simulink subsystem "tireTemp"  (R2022b)
settings: Solver=VariableStepAuto  StartTime=0.0  StopTime=10.0  RelTol=1e-3
libraries: tires x12
settings Model: Creator=serga  LastModifiedBy=serga

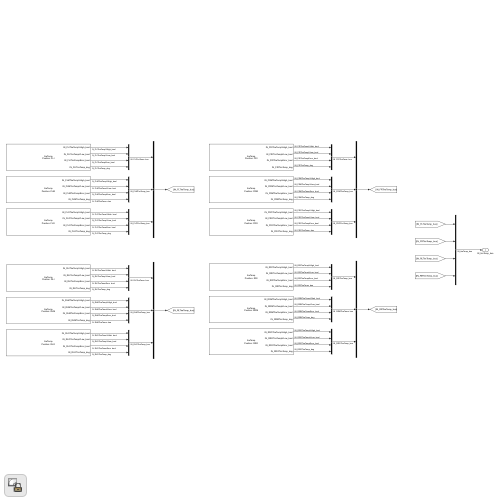
[thumbnail: Simulink's stored preview of the top-level diagram]
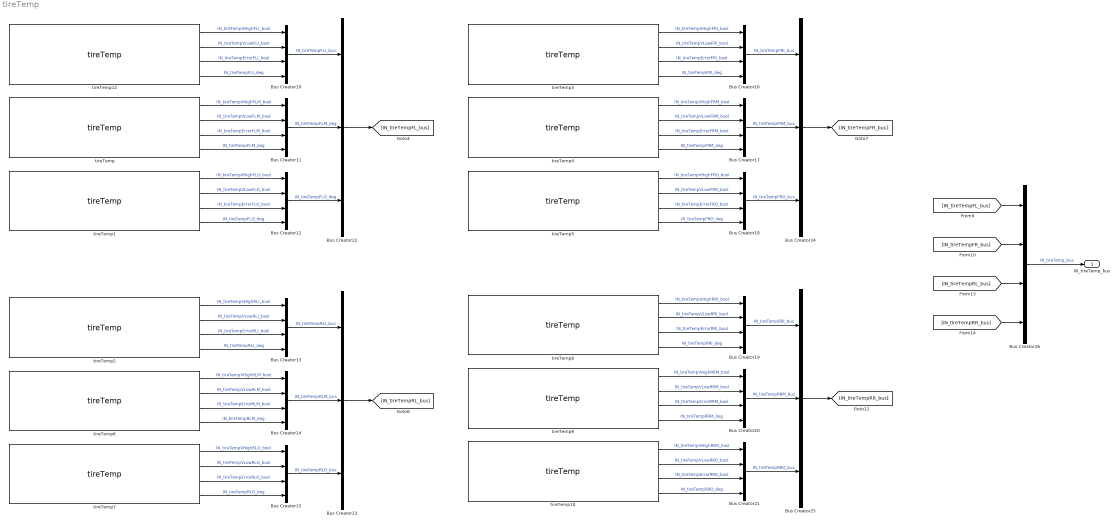
== system tireTemp ==
  Bus Creator{10..21,26} (13 alike) : BusCreator  Inputs=4
  Bus Creator{22..25} (4 alike) : BusCreator  Inputs=3
  tireTemp : tires/tireTemp  pos='FLM'
  tireTemp1 : tires/tireTemp  pos='FLO'
  tireTemp10 : tires/tireTemp  pos='RRO'
  tireTemp12 : tires/tireTemp  pos='FLI'
  tireTemp2 : tires/tireTemp  pos='RLI'
  tireTemp3 : tires/tireTemp  pos='FRI'
  tireTemp4 : tires/tireTemp  pos='FRM'
  tireTemp5 : tires/tireTemp  pos='FRO'
  tireTemp6 : tires/tireTemp  pos='RLM'
  tireTemp7 : tires/tireTemp  pos='RLO'
  tireTemp8 : tires/tireTemp  pos='RRI'
  tireTemp9 : tires/tireTemp  pos='RRM'
  IN_tireTemp_bus : Outport
  wires:
  Bus Creator26/1 -> IN_tireTemp_bus/1  "IN_tireTemp_bus"
  tireTemp2/3 -> Bus Creator13/3  "IN_tireTempErrorRLI_bool"
  tireTemp6/2 -> Bus Creator14/2  "IN_tireTempVLowRLM_bool"
  tireTemp7/4 -> Bus Creator15/4  "IN_tireTempRLO_deg"
  tireTemp3/1 -> Bus Creator16/1  "IN_tireTempVHighFRI_bool"
  tireTemp10/3 -> Bus Creator21/3  "IN_tireTempErrorRRO_bool"
  tireTemp2/1 -> Bus Creator13/1  "IN_tireTempVHighRLI_bool"
  tireTemp7/2 -> Bus Creator15/2  "IN_tireTempVLowRLO_bool"
  tireTemp7/3 -> Bus Creator15/3  "IN_tireTempErrorRLO_bool"
  tireTemp12/2 -> Bus Creator10/2  "IN_tireTempVLowFLI_bool"
  Bus Creator11/1 -> Bus Creator22/2  "IN_tireTempFLM_deg"
  tireTemp4/4 -> Bus Creator17/4  "IN_tireTempFRM_deg"
  [IN_tireTempFL_bus] -> Bus Creator26/1
  tireTemp4/1 -> Bus Creator17/1  "IN_tireTempVHighFRM_bool"
  tireTemp5/2 -> Bus Creator18/2  "IN_tireTempVLowFRO_bool"
  tireTemp6/4 -> Bus Creator14/4  "IN_tireTempRLM_deg"
  tireTemp9/3 -> Bus Creator20/3  "IN_tireTempErrorRRM_bool"
  tireTemp1/1 -> Bus Creator12/1  "IN_tireTempVHighFLO_bool"
  tireTemp10/2 -> Bus Creator21/2  "IN_tireTempVLowRRO_bool"
  tireTemp3/2 -> Bus Creator16/2  "IN_tireTempVLowFRI_bool"
  tireTemp3/4 -> Bus Creator16/4  "IN_tireTempFRI_deg"
  tireTemp12/1 -> Bus Creator10/1  "IN_tireTempVHighFLI_bool"
  tireTemp6/1 -> Bus Creator14/1  "IN_tireTempVHighRLM_bool"
  tireTemp/1 -> Bus Creator11/1  "IN_tireTempVHighFLM_bool"
  tireTemp/2 -> Bus Creator11/2  "IN_tireTempVLowFLM_bool"
  tireTemp12/4 -> Bus Creator10/4  "IN_tireTempFLI_deg"
  tireTemp1/2 -> Bus Creator12/2  "IN_tireTempVLowFLO_bool"
  tireTemp4/2 -> Bus Creator17/2  "IN_tireTempVLowFRM_bool"
  tireTemp1/3 -> Bus Creator12/3  "IN_tireTempErrorFLO_bool"
  tireTemp1/4 -> Bus Creator12/4  "IN_tireTempFLO_deg"
  tireTemp8/2 -> Bus Creator19/2  "IN_tireTempVLowRRI_bool"
  tireTemp2/2 -> Bus Creator13/2  "IN_tireTempVLowRLI_bool"
  tireTemp5/1 -> Bus Creator18/1  "IN_tireTempVHighFRO_bool"
  tireTemp3/3 -> Bus Creator16/3  "IN_tireTempErrorFRI_bool"
  tireTemp10/4 -> Bus Creator21/4  "IN_tireTempRRO_deg"
  Bus Creator10/1 -> Bus Creator22/1  "IN_tireTempFLI_bus"
  Bus Creator21/1 -> Bus Creator25/3  "IN_tireTempRRO_bus"
  tireTemp2/4 -> Bus Creator13/4  "IN_tireTempRLI_deg"
  tireTemp9/2 -> Bus Creator20/2  "IN_tireTempVLowRRM_bool"
  tireTemp9/4 -> Bus Creator20/4  "IN_tireTempRRM_deg"
  Bus Creator24/1 -> [IN_tireTempFR_bus]
  Bus Creator16/1 -> Bus Creator24/1  "IN_tireTempFRI_bus"
  tireTemp/3 -> Bus Creator11/3  "IN_tireTempErrorFLM_bool"
  Bus Creator18/1 -> Bus Creator24/3  "IN_tireTempFRO_bus"
  tireTemp12/3 -> Bus Creator10/3  "IN_tireTempErrorFLI_bool"
  Bus Creator22/1 -> [IN_tireTempFL_bus]
  Bus Creator15/1 -> Bus Creator23/3  "IN_tireTempRLO_bus"
  Bus Creator17/1 -> Bus Creator24/2  "IN_tireTempFRM_bus"
  [IN_tireTempFR_bus] -> Bus Creator26/2
  tireTemp9/1 -> Bus Creator20/1  "IN_tireTempVHighRRM_bool"
  Bus Creator23/1 -> [IN_tireTempRL_bus]
  tireTemp5/4 -> Bus Creator18/4  "IN_tireTempFRO_deg"
  Bus Creator19/1 -> Bus Creator25/1  "IN_tireTempRRI_bus"
  [IN_tireTempRL_bus] -> Bus Creator26/3
  [IN_tireTempRR_bus] -> Bus Creator26/4
  tireTemp5/3 -> Bus Creator18/3  "IN_tireTempErrorFRO_bool"
  Bus Creator14/1 -> Bus Creator23/2  "IN_tireTempRLM_bus"
  Bus Creator20/1 -> Bus Creator25/2  "IN_tireTempRRM_bus"
  tireTemp8/3 -> Bus Creator19/3  "IN_tireTempErrorRRI_bool"
  tireTemp10/1 -> Bus Creator21/1  "IN_tireTempVHighRRO_bool"
  tireTemp7/1 -> Bus Creator15/1  "IN_tireTempVHighRLO_bool"
  tireTemp4/3 -> Bus Creator17/3  "IN_tireTempErrorFRM_bool"
  tireTemp8/4 -> Bus Creator19/4  "IN_tireTempRRI_deg"
  tireTemp8/1 -> Bus Creator19/1  "IN_tireTempVHighRRI_bool"
  Bus Creator25/1 -> [IN_tireTempRR_bus]
  Bus Creator12/1 -> Bus Creator22/3  "IN_tireTempFLO_deg"
  Bus Creator13/1 -> Bus Creator23/1  "IN_tireTempRLI_bus"
  tireTemp/4 -> Bus Creator11/4  "IN_tireTempFLM_deg"
  tireTemp6/3 -> Bus Creator14/3  "IN_tireTempErrorRLM_bool"
